simulink model "Problem1"  (R2020a)
settings: Solver=VariableStepAuto  StartTime=0.0  StopTime=10  RelTol=1e-3
model workspace (MAT data in the model file):
  K1 = 50
  K12 = 10
  M1 = 100
  M2 = 120
  b = 50
settings Model: Creator=kasutav  LastModifiedBy=kasutav

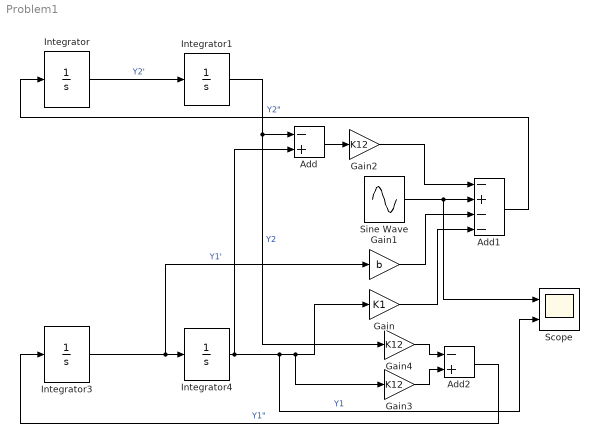
== system Problem1 ==
  Add : Sum  Inputs=-+
  Add1 : Sum  Inputs=-+--
  Add2 : Sum  Inputs=-+
  Gain : Gain  Gain=K1
  Gain1 : Gain  Gain=b
  Gain2 : Gain  Gain=K12
  Gain3 : Gain  Gain=K12
  Gain4 : Gain  Gain=K12
  Integrator{,1,3..4} (4 alike) : Integrator
  Scope : Scope  NumInputPorts=2
  Sine Wave : Sin  Amplitude=2  Frequency=10  SampleTime=0
  wires:
  Add1/1 -> Integrator/1  "Y2\""
  Integrator/1 -> Integrator1/1  "Y2'"
  Integrator1/1 -> Gain4/1, Add/1  "Y2"
  Integrator4/1 -> Add/2, Scope/2, Gain3/1, Gain/1  "Y1"
  Add2/1 -> Integrator3/1  "Y1\""
  Integrator3/1 -> Gain1/1, Integrator4/1  "Y1'"
  Add/1 -> Gain2/1
  Gain2/1 -> Add1/1
  Sine Wave/1 -> Scope/1, Add1/2
  Gain1/1 -> Add1/3
  Gain/1 -> Add1/4
  Gain4/1 -> Add2/1
  Gain3/1 -> Add2/2
